simulink model "CAN_Tranmetter"  (R2021a)
settings: Solver=FixedStepAuto  StartTime=0.0  StopTime=10.0  RelTol=1e-3  EnableMultiTasking=on
libraries: arduinolib x5
settings Model: SILPILModeSetting=veronly  ExtModeTrigDuration=2  Creator=departement-techniqu  LastModifiedBy=departement-techniqu
settings OptimizationCC: EnhancedBackFolding=on  PassReuseOutputArgsAs=Individual arguments  ZeroExternalMemoryAtStartup=off  ZeroInternalMemoryAtStartup=off  MaxStackSize=64  OptimizeBlockOrder=speed  DifferentSizesBufferReuse=on  OptimizationCustomize=off  EfficientTunableParamExpr=on
settings DebuggingCC: ParameterTunabilityLossMsg=error
settings HardwareCC: ProdBitPerInt=16  ProdBitPerPointer=16  ProdBitPerSizeT=16  ProdBitPerPtrDiffT=16  ProdLargestAtomicFloat=None  ProdWordSize=8  ProdHWDeviceType=Atmel->AVR
settings SFSimCC: MATLABDynamicMemAlloc=off
settings RTWCC: SystemTargetFile=ert.tlc  HardwareBoard=Arduino Uno  TemplateMakefile=ert_default_tmf  Toolchain=Arduino AVR  BuildConfiguration=Faster Runs
settings CodeAppCC: ForceParamTrailComments=on  IgnoreCustomStorageClasses=off  OperatorAnnotations=on  SimulinkDataObjDesc=on  SFDataObjDesc=on  InsertBlockDesc=on
settings ERTTargetCC: SupportContinuousTime=on  SupportVariableSizeSignals=on  ExtModeStaticAllocSize=250

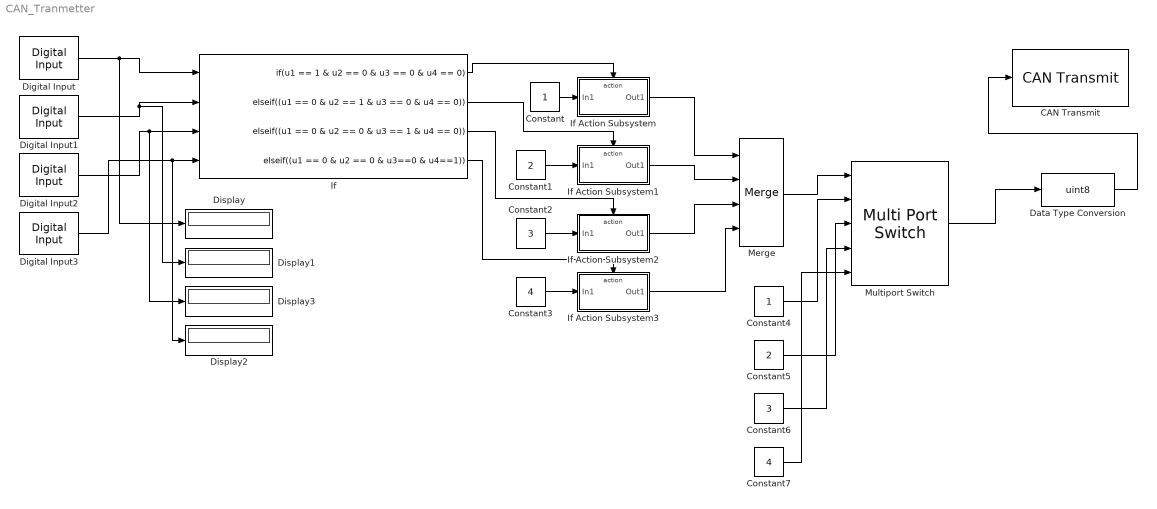
== system CAN_Tranmetter ==
  CAN Transmit : arduinolib/CAN Transmit  inputDataType=Raw data  BlockingMode_=off  BlockTimeout_=1  outputStatus=off  identifierType=Standard (11-bit identifier)  messageId=100  msgLength=1  remoteFrame=off
      settings: SourceProductBaseCode=ARDUINO
  Constant : Constant
  Constant1 : Constant  Value=2
  Constant2 : Constant  Value=3
  Constant3 : Constant  Value=4
  Constant4 : Constant
  Constant5 : Constant  Value=2
  Constant6 : Constant  Value=3
  Constant7 : Constant  Value=4
  Data Type Conversion : DataTypeConversion  OutDataTypeStr=uint8
  Digital Input : arduinolib/Digital Input  pinNumber=1  mode=Default  Direction=input  SampleTime=0.1  blockPlatform=arduino
  Digital Input1 : arduinolib/Digital Input  pinNumber=2  mode=Default  Direction=input  SampleTime=0.1  blockPlatform=arduino
  Digital Input2 : arduinolib/Digital Input  pinNumber=3  mode=Default  Direction=input  SampleTime=0.1  blockPlatform=arduino
  Digital Input3 : arduinolib/Digital Input  pinNumber=4  mode=Default  Direction=input  SampleTime=0.1  blockPlatform=arduino
  Display{,1..3} (4 alike) : Display
  If : If  NumInputs=4  IfExpression=u1 == 1 & u2 == 0 & u3 == 0 & u4 == 0  ElseIfExpressions=(u1 == 0 & u2 == 1 & u3 == 0 & u4 == 0),(u1 == 0 & u2 == 0 & u3 == 1 & u4 == 0),(u1 == 0 & u2 == 0 & u3==0 & u4==1)  ShowElse=off
  If Action Subsystem : Subsystem  TreatAsAtomicUnit=on
  If Action Subsystem1 : Subsystem  TreatAsAtomicUnit=on
  If Action Subsystem2 : Subsystem  TreatAsAtomicUnit=on
  If Action Subsystem3 : Subsystem  TreatAsAtomicUnit=on
  Merge : Merge  Inputs=4
  Multiport Switch : MultiPortSwitch  Inputs=4
  wires:
  If/1 -> If Action Subsystem/Action
  If/2 -> If Action Subsystem1/Action
  If/3 -> If Action Subsystem2/Action
  If/4 -> If Action Subsystem3/Action
  Constant3/1 -> If Action Subsystem3/1(In1)
  Constant2/1 -> If Action Subsystem2/1(In1)
  Constant/1 -> If Action Subsystem/1(In1)
  Constant1/1 -> If Action Subsystem1/1(In1)
  If Action Subsystem/1(Out1) -> Merge/1
  If Action Subsystem1/1(Out1) -> Merge/2
  If Action Subsystem2/1(Out1) -> Merge/3
  If Action Subsystem3/1(Out1) -> Merge/4
  Merge/1 -> Multiport Switch/1
  Constant4/1 -> Multiport Switch/2
  Constant5/1 -> Multiport Switch/3
  Constant6/1 -> Multiport Switch/4
  Constant7/1 -> Multiport Switch/5
  Multiport Switch/1 -> Data Type Conversion/1
  Data Type Conversion/1 -> CAN Transmit/1
  Digital Input/1 -> Display/1, If/1
  Digital Input1/1 -> Display1/1, If/2
  Digital Input2/1 -> Display3/1, If/3
  Digital Input3/1 -> Display2/1, If/4

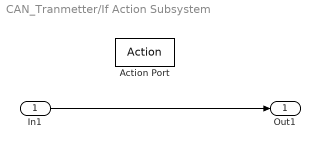
== system CAN_Tranmetter/If Action Subsystem ==
  In1 : Inport
  Action Port : ActionPort  ActionPortLabel=if(u1 == 1 & u2 == 0 & u3 == 0 & u4 == 0)
  Out1 : Outport
  wires:
  In1/1 -> Out1/1

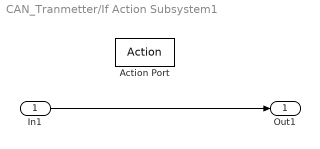
== system CAN_Tranmetter/If Action Subsystem1 ==
  In1 : Inport
  Action Port : ActionPort  ActionPortLabel=elseif((u1 == 0 & u2 == 1 & u3 == 0 & u4 == 0))
  Out1 : Outport
  wires:
  In1/1 -> Out1/1

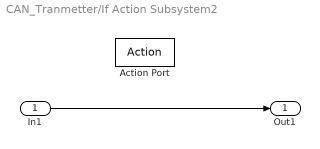
== system CAN_Tranmetter/If Action Subsystem2 ==
  In1 : Inport
  Action Port : ActionPort  ActionPortLabel=elseif((u1 == 0 & u2 == 0 & u3 == 1 & u4 == 0))
  Out1 : Outport
  wires:
  In1/1 -> Out1/1

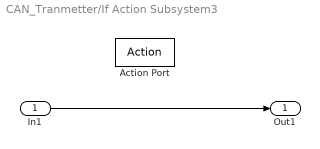
== system CAN_Tranmetter/If Action Subsystem3 ==
  In1 : Inport
  Action Port : ActionPort  ActionPortLabel=elseif((u1 == 0 & u2 == 0 & u3==0 & u4==1))
  Out1 : Outport
  wires:
  In1/1 -> Out1/1
